simulink model "dp2"  (R2017a)
settings: Solver=VariableStepAuto  StartTime=0.0  StopTime=10.0  RelTol=1e-3
undefined symbols (not defined in the file or in its folder): magnitude, xgrid
libraries: simulink x1
settings Model: Creator=thomas  LastModifiedBy=elts2

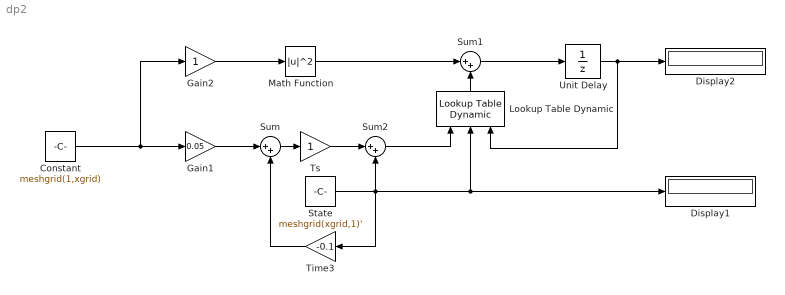
== system dp2 ==
  Constant : Constant  Value=meshgrid(1,xgrid)
  Display1 : Display
  Display2 : Display
  Gain1 : Gain  Gain=0.05
  Gain2 : Gain
  Lookup Table Dynamic : simulink/Lookup Tables/Lookup Table Dynamic  LookUpMeth=Interpolation-Use End Values  OutDataType=fixdt('double')  OutScaling=[]  OutputDataTypeScalingMode=Specify via dialog  OutDataTypeStr=double  DoSatur=off
      settings: SourceProductName=Simulink
  Math Function : Math  Operator=magnitude^2  SaturateOnIntegerOverflow=on
  State : Constant  Value=meshgrid(xgrid,1)'
  Sum : Sum  Inputs=|++
  Sum1 : Sum  Inputs=|++
  Sum2 : Sum  Inputs=|++
  Time3 : Gain  Gain=-0.1
  Ts : Gain
  Unit Delay : UnitDelay  InitialCondition=(1-xgrid).^2
  wires:
  Gain1/1 -> Sum/1
  Gain2/1 -> Math Function/1
  Constant/1 -> Gain1/1, Gain2/1
  Math Function/1 -> Sum1/1
  Sum/1 -> Ts/1
  Time3/1 -> Sum/2
  Unit Delay/1 -> Display2/1, Lookup Table Dynamic/3
  Ts/1 -> Sum2/1
  Sum1/1 -> Unit Delay/1
  Sum2/1 -> Lookup Table Dynamic/1
  Lookup Table Dynamic/1 -> Sum1/2
  State/1 -> Display1/1, Lookup Table Dynamic/2, Sum2/2, Time3/1
